simulink model "gm_untitled"  (R2025a)
settings: Solver=FixedStepDiscrete  StartTime=0.0  StopTime=1000/100000000  RelTol=1e-3
libraries: simulink x1
settings Model: Creator=Luiz  LastModifiedBy=Luiz
settings OptimizationCC: BlockReduction=off  ConditionallyExecuteInputs=off
settings DebuggingCC: InheritedTsInSrcMsg=none

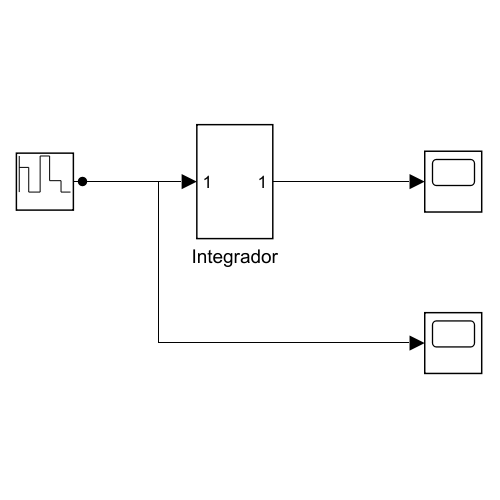
[thumbnail: Simulink's stored preview of the top-level diagram]
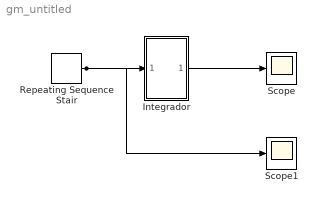
== system gm_untitled ==
  Integrador : Subsystem
  Repeating Sequence Stair : simulink/Sources/Repeating Sequence Stair  OutValues=[3 1 4 2 1].'  tsamp=-1  OutMin=[]  OutMax=[]  OutDataTypeStr=double  OutputDataTypeScalingMode=double  OutDataType=fixdt(0,8)  ConRadixGroup=Best Precision: Vector-wise  OutScaling=2^-12
  Scope : Scope
      settings: ActiveDisplayYMinimum=-5.864285714285722E-7  ActiveDisplayYMaximum=2.5970401785714289E-6
  Scope1 : Scope
      settings: ActiveDisplayYMinimum=0.24568622256738726  ActiveDisplayYMaximum=4.5867799725673883
  wires:
  Integrador/1(Out1) -> Scope/1
  Repeating Sequence Stair/1 -> Integrador/1(In1), Scope1/1

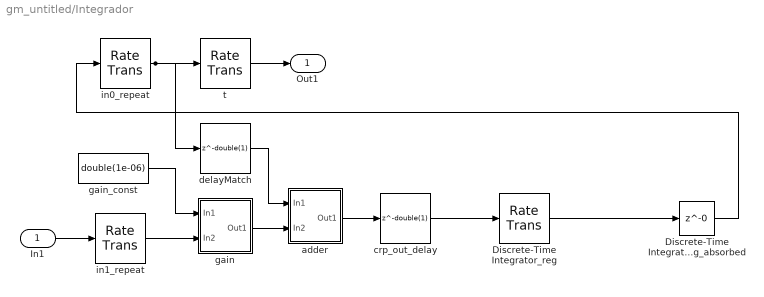
== system gm_untitled/Integrador ==
  In1 : Inport  OutDataTypeStr=double  PortDimensions=1  SampleTime=1e-06
  Discrete-Time Integrator_reg : RateTransition  InitialCondition=double(0)  OutPortSampleTimeOpt=Multiple of input port sample time  OutPortSampleTimeMultiple=100
  Discrete-Time Integrator_reg_absorbed : Delay  DelayLength=0
  adder : Subsystem
      mask Display: disp('NFP\nadd');
  crp_out_delay : Delay  DelayLength=double(1)  InitialCondition=0  SampleTime=1e-08
  delayMatch : Delay  DelayLength=double(1)  InitialCondition=0  SampleTime=1e-08
  gain : Subsystem
      mask Display: disp('NFP\nmul');
  gain_const : Constant  Value=double(1e-06)  OutDataTypeStr=double  SampleTime=1e-08
  in0_repeat : RateTransition  Integrity=off  Deterministic=off  OutPortSampleTimeOpt=Multiple of input port sample time  OutPortSampleTimeMultiple=1/100
  in1_repeat : RateTransition  Integrity=off  Deterministic=off  OutPortSampleTimeOpt=Multiple of input port sample time  OutPortSampleTimeMultiple=1/100
  t : RateTransition  InitialCondition=double(0)  OutPortSampleTimeOpt=Multiple of input port sample time  OutPortSampleTimeMultiple=100
  Out1 : Outport  SampleTime=1e-06
  wires:
  In1/1 -> in1_repeat/1
  in0_repeat/1 -> t/1, delayMatch/1
  gain_const/1 -> gain/1(In1)
  in1_repeat/1 -> gain/2(In2)
  t/1 -> Out1/1
  delayMatch/1 -> adder/1(In1)
  gain/1(Out1) -> adder/2(In2)
  adder/1(Out1) -> crp_out_delay/1
  crp_out_delay/1 -> Discrete-Time Integrator_reg/1
  Discrete-Time Integrator_reg/1 -> Discrete-Time Integrator_reg_absorbed/1
  Discrete-Time Integrator_reg_absorbed/1 -> in0_repeat/1

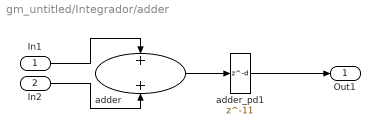
== system gm_untitled/Integrador/adder ==
  In1 : Inport
  In2 : Inport  Port=2
  adder : Sum  OutDataTypeStr=double  SampleTime=1e-08
  adder_pd1 : Delay  DelayLength=11
  Out1 : Outport
  wires:
  In1/1 -> adder/1
  In2/1 -> adder/2
  adder/1 -> adder_pd1/1
  adder_pd1/1 -> Out1/1

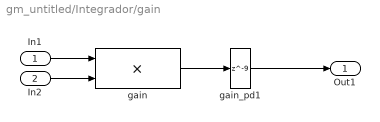
== system gm_untitled/Integrador/gain ==
  In1 : Inport
  In2 : Inport  Port=2
  gain : Product  Inputs=**  OutDataTypeStr=double  SampleTime=1e-08
  gain_pd1 : Delay  DelayLength=9
  Out1 : Outport
  wires:
  In1/1 -> gain/1
  In2/1 -> gain/2
  gain/1 -> gain_pd1/1
  gain_pd1/1 -> Out1/1
